simulink subsystem "Bits_Colision"  (R2024b)
settings: Solver=VariableStepAuto  StartTime=0.0  StopTime=10.0  RelTol=1e-3
libraries: arduinosensorlib x4
settings Model: Creator=Chenfu  LastModifiedBy=Chenfu

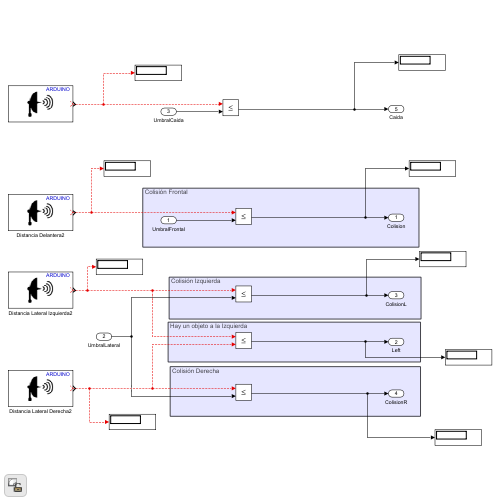
[thumbnail: Simulink's stored preview of the top-level diagram]
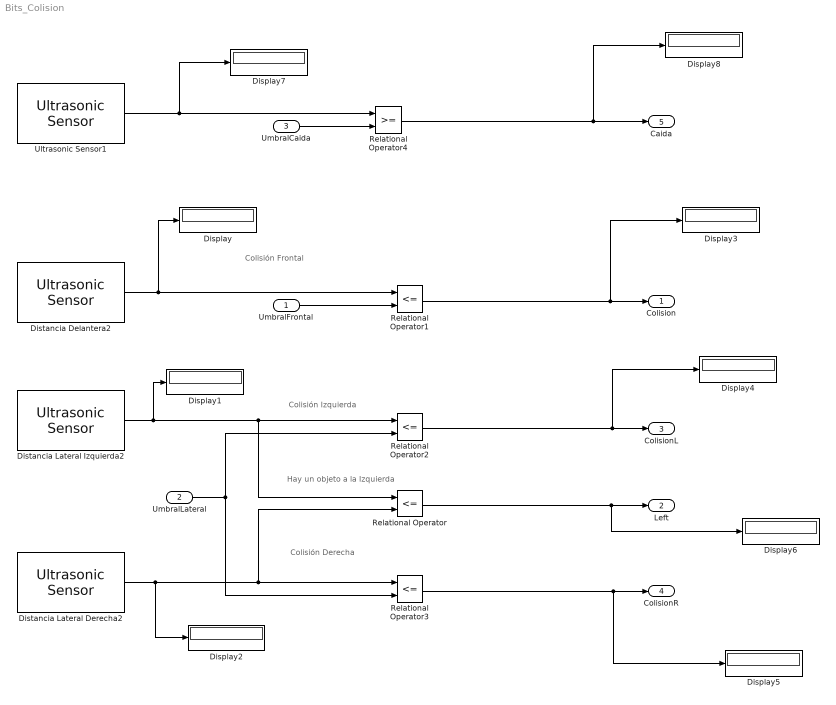
== system Bits_Colision ==
  note: Colisión Derecha
  note: Hay un objeto a la Izquierda
  note: Colisión Izquierda
  note: Colisión Frontal
  UmbralFrontal : Inport
  UmbralLateral : Inport  Port=2
  UmbralCaida : Inport  Port=3
  Display{,1..8} (9 alike) : Display
  Distancia Delantera2 : arduinosensorlib/Ultrasonic Sensor  NumSignalPins=2  TrigPin=9  EchoPin=8  SignalPin=3  SampleTime_=0.1  blockPlatform=ARDUINO
  Distancia Lateral Derecha2 : arduinosensorlib/Ultrasonic Sensor  NumSignalPins=2  TrigPin=11  EchoPin=10  SignalPin=3  SampleTime_=0.1  blockPlatform=ARDUINO
  Distancia Lateral Izquierda2 : arduinosensorlib/Ultrasonic Sensor  NumSignalPins=2  TrigPin=13  EchoPin=12  SignalPin=3  SampleTime_=0.1  blockPlatform=ARDUINO
  Relational Operator{,1..3} (4 alike) : RelationalOperator  Operator=<=  OutDataTypeStr=boolean  RndMeth=Simplest  InputSameDT=off
  Relational Operator4 : RelationalOperator  OutDataTypeStr=boolean  RndMeth=Simplest  InputSameDT=off
  Ultrasonic Sensor1 : arduinosensorlib/Ultrasonic Sensor  NumSignalPins=2  TrigPin=7  EchoPin=6  SignalPin=3  SampleTime_=0.1  blockPlatform=ARDUINO
  Colision : Outport
  Left : Outport  Port=2
  ColisionL : Outport  Port=3
  ColisionR : Outport  Port=4
  Caida : Outport  Port=5
  wires:
  Relational Operator/1 -> Left/1, Display6/1
  Distancia Delantera2/1 -> Relational Operator1/1, Display/1
  UmbralFrontal/1 -> Relational Operator1/2
  Relational Operator1/1 -> Colision/1, Display3/1
  Distancia Lateral Izquierda2/1 -> Relational Operator/1, Relational Operator2/1, Display1/1
  Distancia Lateral Derecha2/1 -> Relational Operator/2, Relational Operator3/1, Display2/1
  UmbralLateral/1 -> Relational Operator2/2, Relational Operator3/2
  Relational Operator2/1 -> ColisionL/1, Display4/1
  Relational Operator3/1 -> ColisionR/1, Display5/1
  Ultrasonic Sensor1/1 -> Display7/1, Relational Operator4/1
  UmbralCaida/1 -> Relational Operator4/2
  Relational Operator4/1 -> Caida/1, Display8/1
